simulink model "ass4_fin"  (R2023b)
settings: Solver=VariableStepAuto  StartTime=0.0  StopTime=100  RelTol=1e-3
undefined symbols (not defined in the file): DiscIntNeverNeededParam
libraries: dspstat3 x12, dspadpt3 x8, fuzblock x3, dspsrcs4 x2
settings Model: Creator=Aditya Prachand  LastModifiedBy=Asus

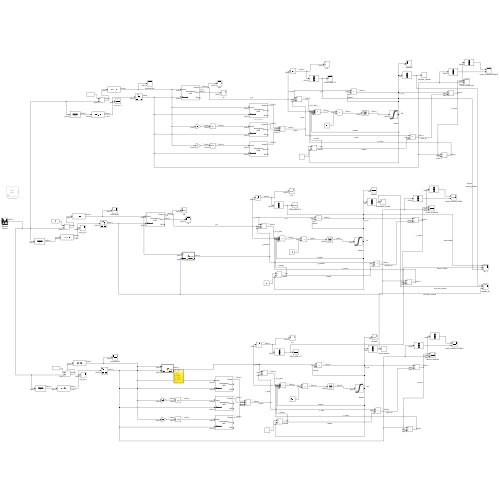
[thumbnail: Simulink's stored preview of the top-level diagram]
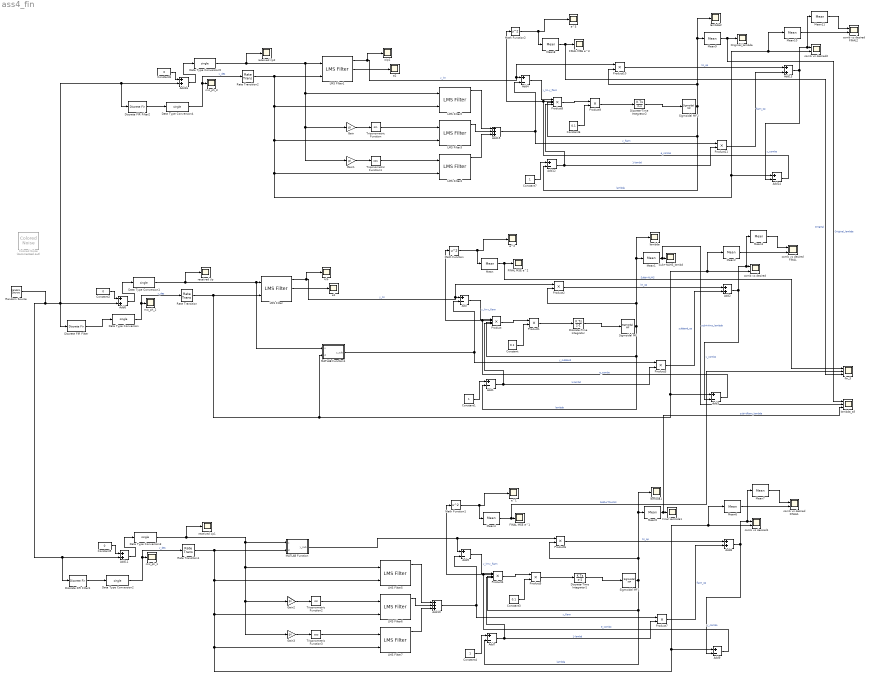
== system ass4_fin ==
  Add{,1,3..5,7,9,12,14} (9 alike) : Sum  Inputs=+-
  Add10 : Sum  Inputs=+++
  Add{2,6,8,11,13,16} (6 alike) : Sum
  Add15 : Sum  Inputs=+++
  Colored Noise : dspsrcs4/Colored Noise  Commented=on  Color=pink  InverseFrequencyPower=1  BoundedOutput=on  NumChannels=1  OutputDataType=double  SamplesPerFrame=255  SampleTime=1/16000  RandomStream=mt19937ar with seed  Seed=67  SimulateUsing=Interpreted execution
      settings: LibrarySourceBlock=audiosources/Colored Noise
  Constant : Constant  Value=0.1
  Constant1 : Constant
  Constant2 : Constant  Value=0  OutDataTypeStr=single
  Constant3 : Constant  Value=0.1
  Constant4 : Constant
  Constant5 : Constant  Value=0  OutDataTypeStr=single
  Constant6 : Constant  Value=0.1
  Constant7 : Constant
  Constant8 : Constant  Value=0  OutDataTypeStr=single
  Data Type Conversion{,1..5} (6 alike) : DataTypeConversion  OutDataTypeStr=single  SaturateOnIntegerOverflow=off  RndMeth=Floor
  Discrete FIR Filter : DiscreteFir  Coefficients=[1, 0.5, -0.2, 0.1, -0.05]  InputProcessing=Columns as channels (frame based)
  Discrete FIR Filter1 : DiscreteFir  Coefficients=[1, 0.5, -0.2, 0.1, -0.05]  InputProcessing=Columns as channels (frame based)
  Discrete FIR Filter2 : DiscreteFir  Coefficients=[1, 0.5, -0.2, 0.1, -0.05]  InputProcessing=Columns as channels (frame based)
  Discrete-Time Integrator : DiscreteIntegrator  SampleTime=-1  ICPrevOutput=DiscIntNeverNeededParam  ICPrevScaledInput=DiscIntNeverNeededParam
  Discrete-Time Integrator1 : DiscreteIntegrator  SampleTime=-1  ICPrevOutput=DiscIntNeverNeededParam  ICPrevScaledInput=DiscIntNeverNeededParam
  Discrete-Time Integrator2 : DiscreteIntegrator  SampleTime=-1  ICPrevOutput=DiscIntNeverNeededParam  ICPrevScaledInput=DiscIntNeverNeededParam
  FINAL MSE e^1 : Scope
  FINAL MSE e^2 : Scope
  FINAL MSE e^3 : Scope
  Final Lambda1 : Scope
  Gain{,1..3} (4 alike) : Gain  Gain=pi
  LMS Filter : dspadpt3/LMS Filter  Algo=Normalized LMS  L=4  stepflag=Dialog  mu=0.1  leakage=1.0  ic=0  Adapt=off  resetflag=None  weights=on  addnparflag=off  roundingMode=Floor  overflowMode=on  firstCoeffMode=Specify word length  firstCoeffWordLength=16  firstCoeffFracLength=15
  LMS Filter1 : dspadpt3/LMS Filter  Algo=Normalized LMS  L=4  stepflag=Dialog  mu=0.1  leakage=1.0  ic=0  Adapt=off  resetflag=None  weights=on  addnparflag=off  roundingMode=Floor  overflowMode=on  firstCoeffMode=Specify word length  firstCoeffWordLength=16  firstCoeffFracLength=15
  LMS Filter{2..7} (6 alike) : dspadpt3/LMS Filter  Algo=Normalized LMS  L=96  stepflag=Dialog  mu=0.001  leakage=1.0  ic=0  Adapt=off  resetflag=None  weights=on  addnparflag=off  roundingMode=Floor  overflowMode=off
  MATLAB Function : MATLAB Function  TreatAsAtomicUnit=on
  MATLAB Function1 : MATLAB Function  TreatAsAtomicUnit=on
  Math Function : Math  Operator=square
  Math Function1 : Math  Operator=square
  Math Function2 : Math  Operator=square
  Mean{,1..11} (12 alike) : dspstat3/Mean  run=off  InputProcessing=Columns as channels (frame based)  reset_popup=None  directionMode=Entire input  dimension=1  roiEnable=off  roiType=Rectangles  roiPortion=Entire ROI  roiOutput=Individual statistics for each ROI  roiFlag=off  roundingMode=Floor  overflowMode=off  outputDataTypeStr=Inherit: Same as accumulator  outputMin=[]  outputMax=[]  outputLastDataTypeStr=Inherit: Same as accumulator
  Originial_lambda : Scope
  Product : Product  Inputs=4
  Product{1..3,5..7,9..11} (9 alike) : Product
  Product4 : Product  Inputs=4
  Product8 : Product  Inputs=4
  Random Source : dspsrcs4/Random Source  SrcType=Gaussian  NormMethod=Ziggurat  CltLength=12  MinVal=0  MaxVal=1  MeanVal=0  VarVal=1  RepMode=Not repeatable  rawSeed=1  IsInherit=off  SampMode=Discrete  SampTime=1/16000  SampFrame=255  DataType=Single  OutComplex=Real  OutputFrames=off
  Rate Transition : RateTransition  Integrity=off  OutPortSampleTimeOpt=Inherit
  Rate Transition1 : RateTransition  Integrity=off  OutPortSampleTimeOpt=Inherit
  Rate Transition2 : RateTransition  Integrity=off  OutPortSampleTimeOpt=Inherit
  Sigmoidal MF : fuzblock/Membership  Functions/Sigmoidal MF  a=1  c=0
  Sigmoidal MF1 : fuzblock/Membership  Functions/Sigmoidal MF  a=1  c=0
  Sigmoidal MF2 : fuzblock/Membership  Functions/Sigmoidal MF  a=1  c=0
  Sub+NLMS_lambd : Scope
  Trigonometric Function : Trigonometry
  Trigonometric Function1 : Trigonometry  Operator=cos
  Trigonometric Function2 : Trigonometry
  Trigonometric Function3 : Trigonometry  Operator=cos
  comb vs desired : Scope  NumInputPorts=2
  comb vs desired FINAL : Scope  NumInputPorts=2
  comb vs desired FINAL1 : Scope  NumInputPorts=2
  comb vs desired FINAL2 : Scope  NumInputPorts=2
  comb vs desired1 : Scope  NumInputPorts=2
  comb vs desired2 : Scope  NumInputPorts=2
  e1 : Scope
  e2 : Scope
  e^1 : Scope
  e^2 : Scope
  e^3 : Scope
  fin_3 : Scope  NumInputPorts=3
  lambda : Scope
  lambda1 : Scope
  lambda2 : Scope
  lambda_all : Scope  NumInputPorts=3
  mic_ph_1 : Scope
  mic_ph_2 : Scope
  mic_ph_3 : Scope
  o/p : Scope
  o/p1 : Scope
  received i/p : Scope
  received i/p1 : Scope
  received i/p2 : Scope
  wires:
  Product1/1 -> Discrete-Time Integrator/1
  Constant/1 -> Product1/2
  Data Type Conversion1/1 -> MATLAB Function1/1(x), LMS Filter/1, received i/p/1
  LMS Filter/2 -> e1/1
  Mean2/1 -> comb vs desired FINAL/2
  Mean1/1 -> lambda_all/2, Sub+NLMS_lambd/1  "sub+nlms_lambda"
  Rate Transition/1 -> LMS Filter/2, MATLAB Function1/2(d), Add3/1, Mean2/1, comb vs desired/2
  Math Function/1 -> Mean/1, e^2/1
  Add/1 -> Product/1  "y_lin-y_flann"
  Constant1/1 -> Add1/1
  Constant2/1 -> Add6/1
  Add3/1 -> Math Function/1, Product/2  "e_combo"
  MATLAB Function1/1(y_sub) -> Add/2, Product3/1  "y_subband"
  Add2/1 -> Mean3/1, comb vs desired/1, Add3/2  "y_combo"
  LMS Filter/1 -> Product2/1, Add/1, o/p/1  "y_lin"
  Data Type Conversion/1 -> mic_ph_2/1, Rate Transition/1  "y_des"
  Add1/1 -> Product/4, Product3/2  "1-lambd"
  Discrete-Time Integrator/1 -> Sigmoidal MF/1
  Mean/1 -> fin_3/1, FINAL MSE e^2/1  "Subb+NLMS"
  Mean3/1 -> comb vs desired FINAL/1
  Sigmoidal MF/1 -> Mean1/1, lambda/1, Product2/2, Add1/2, Product/3  "lambda"
  Product/1 -> Product1/1
  Product2/1 -> Add2/1  "lin_op"
  Add6/1 -> Data Type Conversion1/1
  Discrete FIR Filter/1 -> Data Type Conversion/1
  Product3/1 -> Add2/2  "subband_op"
  MATLAB Function/1(y_sub) -> Add5/1, Product6/1
  Product5/1 -> Discrete-Time Integrator1/1
  Rate Transition1/1 -> MATLAB Function/2(d), Add9/1, Mean6/1, comb vs desired1/2, LMS Filter7/2, LMS Filter6/2, LMS Filter5/2
  Data Type Conversion3/1 -> MATLAB Function/1(x), LMS Filter5/1, Gain3/1, Gain2/1, received i/p1/1
  Gain3/1 -> Trigonometric Function3/1
  Mean5/1 -> lambda_all/3, Final Lambda1/1  "sub+tflann_lambda"
  Sigmoidal MF1/1 -> Mean5/1, lambda1/1, Product6/2, Add7/2, Product4/3  "lambda"
  Mean6/1 -> comb vs desired FINAL1/2
  Product4/1 -> Product5/1
  Constant3/1 -> Product5/2
  Trigonometric Function3/1 -> LMS Filter7/1
  Gain2/1 -> Trigonometric Function2/1
  Add5/1 -> Product4/1  "y_lin-y_flann"
  Add7/1 -> Product4/4, Product7/2  "1-lambd"
  LMS Filter7/1 -> Add10/3
  Math Function1/1 -> Mean4/1, e^1/1
  LMS Filter6/1 -> Add10/2
  Constant5/1 -> Add11/1
  Discrete-Time Integrator1/1 -> Sigmoidal MF1/1
  Add8/1 -> Mean7/1, comb vs desired1/1, Add9/2  "y_combo"
  Mean4/1 -> fin_3/2, FINAL MSE e^1/1  "Subb+TFLANN"
  Discrete FIR Filter1/1 -> Data Type Conversion2/1
  Data Type Conversion2/1 -> mic_ph_1/1, Rate Transition1/1  "y_des"
  Constant4/1 -> Add7/1
  Trigonometric Function2/1 -> LMS Filter6/1
  Add9/1 -> Math Function1/1, Product4/2  "e_combo"
  Add11/1 -> Data Type Conversion3/1
  LMS Filter5/1 -> Add10/1
  Product6/1 -> Add8/1  "lin_op"
  Add10/1 -> Add5/2, Product7/1  "y_flann"
  Mean7/1 -> comb vs desired FINAL1/1
  Random Source/1 -> Add11/2, Discrete FIR Filter1/1, Add6/2, Discrete FIR Filter/1, Add16/2, Discrete FIR Filter2/1
  Product7/1 -> Add8/2  "flann_op"
  Sigmoidal MF2/1 -> Mean9/1, lambda2/1, Product10/2, Add12/2, Product8/3  "lambda"
  Product9/1 -> Discrete-Time Integrator2/1
  Discrete-Time Integrator2/1 -> Sigmoidal MF2/1
  Add15/1 -> Add4/2, Product11/1  "y_flann"
  Rate Transition2/1 -> LMS Filter1/2, Add14/1, Mean10/1, comb vs desired2/2, LMS Filter4/2, LMS Filter3/2, LMS Filter2/2
  Math Function2/1 -> Mean8/1, e^3/1
  Product11/1 -> Add13/2  "flann_op"
  Add16/1 -> Data Type Conversion5/1
  Constant8/1 -> Add16/1
  Add14/1 -> Math Function2/1, Product8/2  "e_combo"
  Discrete FIR Filter2/1 -> Data Type Conversion4/1
  LMS Filter1/2 -> e2/1
  Product8/1 -> Product9/1
  LMS Filter4/1 -> Add15/3
  Product10/1 -> Add13/1  "lin_op"
  Add12/1 -> Product8/4, Product11/2  "1-lambd"
  Mean8/1 -> fin_3/3, FINAL MSE e^3/1  "Original"
  Data Type Conversion4/1 -> mic_ph_3/1, Rate Transition2/1  "y_des"
  Mean10/1 -> comb vs desired FINAL2/2
  Constant6/1 -> Product9/2
  Constant7/1 -> Add12/1
  Trigonometric Function/1 -> LMS Filter3/1
  Gain/1 -> Trigonometric Function/1
  LMS Filter3/1 -> Add15/2
  Mean11/1 -> comb vs desired FINAL2/1
  Add13/1 -> Mean11/1, comb vs desired2/1, Add14/2  "y_combo"
  Data Type Conversion5/1 -> LMS Filter1/1, LMS Filter2/1, Gain1/1, Gain/1, received i/p2/1
  Mean9/1 -> lambda_all/1, Originial_lambda/1  "Original_lambda"
  LMS Filter2/1 -> Add15/1
  Add4/1 -> Product8/1  "y_lin-y_flann"
  Trigonometric Function1/1 -> LMS Filter4/1
  Gain1/1 -> Trigonometric Function1/1
  LMS Filter1/1 -> Product10/1, Add4/1, o/p1/1  "y_lin"

== matlab function ass4_fin/MATLAB Function ==
  data: x input; y_sub output; d input
function y_sub = subband_6band_filter(x, d)
% Inputs: x (frame/sample of reference signal), d (frame/sample of desired signal)
% Output: y_sub (estimated linear output)

% Store the original data type to prevent Simulink type-mismatch errors
original_type = class(x);

% Cast inputs to 'double' for precise computation
x = double(x);
d = double(d);

frame_size = length(x);
y_sub_double = zeros(frame_size, 1);

% Persistent variables retain state across Simulink time steps
persistent W X_buffer D_buffer x_band_buffer H K L mu Order

% Initialization (Runs only on the first simulation step)
if isempty(W)
    K = 6;              % Number of subbands
    L = 32;             % Taps per subband filter
    mu = 0.005;         % Step size (tune carefully)
    Order = 48;         % Analysis filter bank order
    
    W = zeros(L, K);
    X_buffer = zeros(Order + 1, 1);
    D_buffer = zeros(Order + 1, 1);
    x_band_buffer = zeros(L, K);
    H = zeros(Order + 1, K);
    
    % Design the 6-Band Filter Bank
    for k = 1:K
        f_low = (k - 1) / K;
        f_high = k / K;
        
        if k == 1
            H(:, k) = fir1(Order, f_high, 'low')';
        elseif k == K
            H(:, k) = fir1(Order, f_low, 'high')';
        else
            H(:, k) = fir1(Order, [f_low, f_high], 'bandpass')';
        end
    end
end

% Process the incoming frame sample-by-sample
for i = 1:frame_size
    
    x_in = x(i);
    d_in = d(i);

    % 1. Update Filter Bank Delay Lines
    X_buffer = [x_in; X_buffer(1:end-1)];
    D_buffer = [d_in; D_buffer(1:end-1)];

    y_out_sample = 0; % Accumulator for the combined output
    
    % 2. Process each of the 6 subbands
    for k = 1:K
        % Split signals into current band
        x_k = sum(H(:, k) .* X_buffer); 
        d_k = sum(H(:, k) .* D_buffer); 
        
        % Update Adaptive Filter Delay Line for band k
        x_band_buffer(:, k) = [x_k; x_band_buffer(1:end-1, k)];
        
        % Subband Output and Error Calculation
        y_k = W(:, k)' * x_band_buffer(:, k);
        e_k = d_k - y_k;
        
        % Subband Weight Update (LMS)
        W(:, k) = W(:, k) + mu * e_k * x_band_buffer(:, k);
        
        % Accumulate the synthesis output
        y_out_sample = y_out_sample + y_k;
    end
    
    % Store the synthesized full-band sample
    y_sub_double(i) = y_out_sample;
end

% Cast the final output back to the original type for downstream blocks
y_sub = cast(y_sub_double, original_type);

end

== matlab function ass4_fin/MATLAB Function1 ==
  data: x input; y_sub output; d input
function y_sub = subband_6band_filter(x, d)
% Inputs: x (frame/sample of reference signal), d (frame/sample of desired signal)
% Output: y_sub (estimated linear output)

% Store the original data type to prevent Simulink type-mismatch errors
original_type = class(x);

% Cast inputs to 'double' for precise computation
x = double(x);
d = double(d);

frame_size = length(x);
y_sub_double = zeros(frame_size, 1);

% Persistent variables retain state across Simulink time steps
persistent W X_buffer D_buffer x_band_buffer H K L mu Order

% Initialization (Runs only on the first simulation step)
if isempty(W)
    K = 6;              % Number of subbands
    L = 32;             % Taps per subband filter
    mu = 0.005;         % Step size (tune carefully)
    Order = 48;         % Analysis filter bank order
    
    W = zeros(L, K);
    X_buffer = zeros(Order + 1, 1);
    D_buffer = zeros(Order + 1, 1);
    x_band_buffer = zeros(L, K);
    H = zeros(Order + 1, K);
    
    % Design the 6-Band Filter Bank
    for k = 1:K
        f_low = (k - 1) / K;
        f_high = k / K;
        
        if k == 1
            H(:, k) = fir1(Order, f_high, 'low')';
        elseif k == K
            H(:, k) = fir1(Order, f_low, 'high')';
        else
            H(:, k) = fir1(Order, [f_low, f_high], 'bandpass')';
        end
    end
end

% Process the incoming frame sample-by-sample
for i = 1:frame_size
    
    x_in = x(i);
    d_in = d(i);

    % 1. Update Filter Bank Delay Lines
    X_buffer = [x_in; X_buffer(1:end-1)];
    D_buffer = [d_in; D_buffer(1:end-1)];

    y_out_sample = 0; % Accumulator for the combined output
    
    % 2. Process each of the 6 subbands
    for k = 1:K
        % Split signals into current band
        x_k = sum(H(:, k) .* X_buffer); 
        d_k = sum(H(:, k) .* D_buffer); 
        
        % Update Adaptive Filter Delay Line for band k
        x_band_buffer(:, k) = [x_k; x_band_buffer(1:end-1, k)];
        
        % Subband Output and Error Calculation
        y_k = W(:, k)' * x_band_buffer(:, k);
        e_k = d_k - y_k;
        
        % Subband Weight Update (LMS)
        W(:, k) = W(:, k) + mu * e_k * x_band_buffer(:, k);
        
        % Accumulate the synthesis output
        y_out_sample = y_out_sample + y_k;
    end
    
    % Store the synthesized full-band sample
    y_sub_double(i) = y_out_sample;
end

% Cast the final output back to the original type for downstream blocks
y_sub = cast(y_sub_double, original_type);

end
